simulink model "PID_finder"  (R2022b)
settings: Solver=ode4  StartTime=0.0  StopTime=30  FixedStep=0.02  RelTol=1e-3
undefined symbols (not defined in the file or in its folder): DiscIntNeverNeededParam, LQIDG_openloop_pitch, LQIDG_openloop_pitch_d, LQIDG_openloop_roll, LQIDG_openloop_roll_d
libraries: simulink_extras x2, slpidlib x2
settings Model: Creator=Ali  LastModifiedBy=Ali

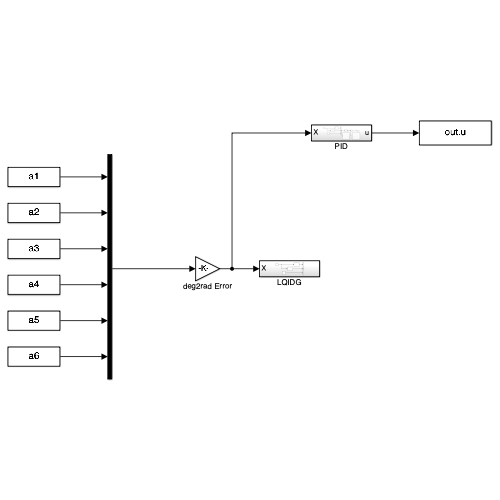
[thumbnail: Simulink's stored preview of the top-level diagram]
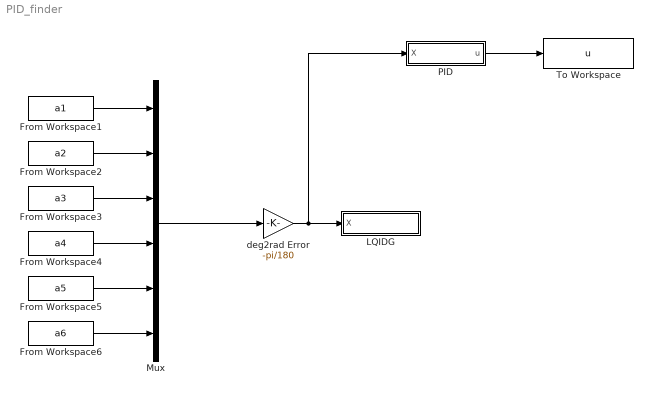
== system PID_finder ==
  From Workspace1 : FromWorkspace  VariableName=a1
  From Workspace2 : FromWorkspace  VariableName=a2
  From Workspace3 : FromWorkspace  VariableName=a3
  From Workspace4 : FromWorkspace  VariableName=a4
  From Workspace5 : FromWorkspace  VariableName=a5
  From Workspace6 : FromWorkspace  VariableName=a6
  LQIDG : Subsystem
  Mux : Mux  Inputs=6
  PID : Subsystem
  To Workspace : ToWorkspace  VariableName=u  SaveFormat=Timeseries  SampleTime=-1
  deg2rad Error : Gain  Gain=-pi/180
  wires:
  deg2rad Error/1 -> PID/1(X), LQIDG/1(X)
  Mux/1 -> deg2rad Error/1
  From Workspace1/1 -> Mux/1
  From Workspace3/1 -> Mux/3
  From Workspace2/1 -> Mux/2
  From Workspace4/1 -> Mux/4
  From Workspace5/1 -> Mux/5
  From Workspace6/1 -> Mux/6
  PID/1(u) -> To Workspace/1

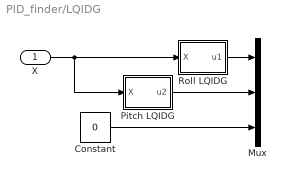
== system PID_finder/LQIDG ==
  X : Inport
  Constant : Constant  Value=0
  Mux : Mux  Inputs=3
  Pitch LQIDG : Subsystem
  Roll LQIDG : Subsystem
  wires:
  Constant/1 -> Mux/3
  Pitch LQIDG/1(u2) -> Mux/2
  X/1 -> Pitch LQIDG/1(X), Roll LQIDG/1(X)
  Roll LQIDG/1(u1) -> Mux/1

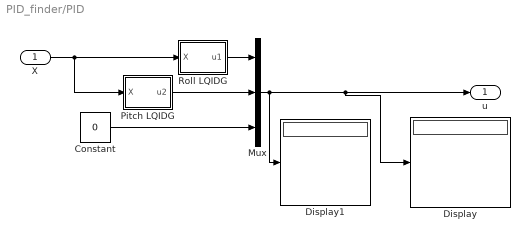
== system PID_finder/PID ==
  X : Inport
  Constant : Constant  Value=0
  Display : Display
  Display1 : Display
  Mux : Mux  Inputs=3
  Pitch LQIDG : Subsystem
  Roll LQIDG : Subsystem
  u : Outport
  wires:
  Mux/1 -> u/1, Display/1, Display1/1
  Constant/1 -> Mux/3
  Pitch LQIDG/1(u2) -> Mux/2
  X/1 -> Pitch LQIDG/1(X), Roll LQIDG/1(X)
  Roll LQIDG/1(u1) -> Mux/1

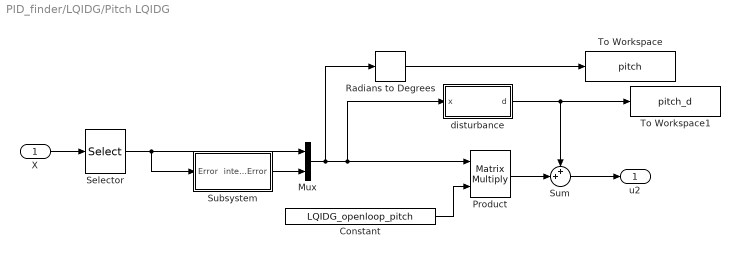
== system PID_finder/LQIDG/Pitch LQIDG ==
  X : Inport
  Constant : Constant  Value=LQIDG_openloop_pitch
  Mux : Mux  Inputs=2
  Product : Product  Multiplication=Matrix(*)
  Radians to Degrees : simulink_extras/Transformations/Radians to Degrees
  Selector : Selector  InputPortWidth=6  IndexOptions=Index vector (dialog)  Indices=[2 5]  OutputSizes=1
  Subsystem : Subsystem
  Sum : Sum  Inputs=++|
  To Workspace : ToWorkspace  VariableName=pitch  SaveFormat=Timeseries  SampleTime=-1
  To Workspace1 : ToWorkspace  VariableName=pitch_d  SaveFormat=Timeseries  SampleTime=-1
  disturbance : Subsystem
  u2 : Outport
  wires:
  Constant/1 -> Product/2
  X/1 -> Selector/1
  Subsystem/1(integ_Error) -> Mux/2
  Selector/1 -> Subsystem/1(Error), Mux/1
  Mux/1 -> Radians to Degrees/1, disturbance/1(x), Product/1
  disturbance/1(d) -> Sum/1, To Workspace1/1
  Product/1 -> Sum/2
  Sum/1 -> u2/1
  Radians to Degrees/1 -> To Workspace/1

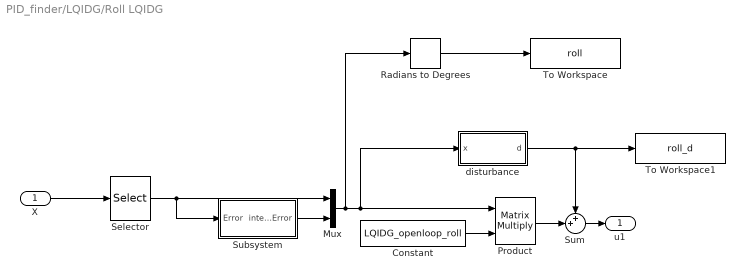
== system PID_finder/LQIDG/Roll LQIDG ==
  X : Inport
  Constant : Constant  Value=LQIDG_openloop_roll
  Mux : Mux  Inputs=2
  Product : Product  Multiplication=Matrix(*)
  Radians to Degrees : simulink_extras/Transformations/Radians to Degrees
  Selector : Selector  InputPortWidth=6  IndexOptions=Index vector (dialog)  Indices=[1 4]  OutputSizes=1
  Subsystem : Subsystem
  Sum : Sum  Inputs=++|
  To Workspace : ToWorkspace  VariableName=roll  SaveFormat=Timeseries  SampleTime=-1
  To Workspace1 : ToWorkspace  VariableName=roll_d  SaveFormat=Timeseries  SampleTime=-1
  disturbance : Subsystem
  u1 : Outport
  wires:
  Constant/1 -> Product/2
  Mux/1 -> Radians to Degrees/1, disturbance/1(x), Product/1
  X/1 -> Selector/1
  Subsystem/1(integ_Error) -> Mux/2
  Selector/1 -> Subsystem/1(Error), Mux/1
  Product/1 -> Sum/2
  Sum/1 -> u1/1
  disturbance/1(d) -> Sum/1, To Workspace1/1
  Radians to Degrees/1 -> To Workspace/1

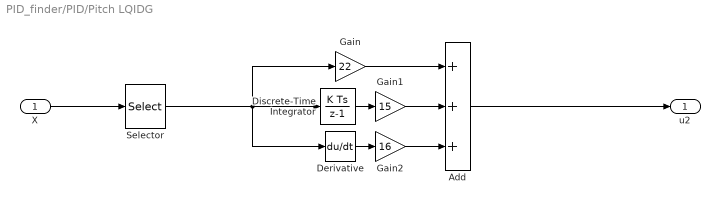
== system PID_finder/PID/Pitch LQIDG ==
  X : Inport
  Add : Sum  Inputs=+++
  Derivative : Derivative
  Discrete-Time Integrator : DiscreteIntegrator  SampleTime=-1  ICPrevOutput=DiscIntNeverNeededParam  ICPrevScaledInput=DiscIntNeverNeededParam
  Gain : Gain  Gain=22
  Gain1 : Gain  Gain=15
  Gain2 : Gain  Gain=16
  Selector : Selector  InputPortWidth=6  IndexOptions=Index vector (dialog)  Indices=[2]  OutputSizes=1
  u2 : Outport
  wires:
  X/1 -> Selector/1
  Selector/1 -> Discrete-Time Integrator/1, Gain/1, Derivative/1
  Gain1/1 -> Add/2
  Gain2/1 -> Add/3
  Discrete-Time Integrator/1 -> Gain1/1
  Derivative/1 -> Gain2/1
  Gain/1 -> Add/1
  Add/1 -> u2/1

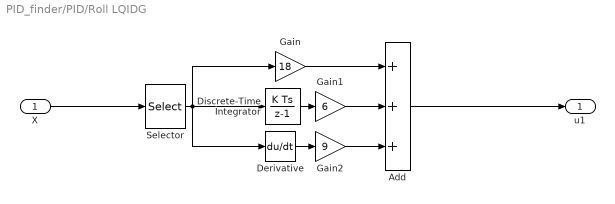
== system PID_finder/PID/Roll LQIDG ==
  X : Inport
  Add : Sum  Inputs=+++
  Derivative : Derivative
  Discrete-Time Integrator : DiscreteIntegrator  SampleTime=-1  ICPrevOutput=DiscIntNeverNeededParam  ICPrevScaledInput=DiscIntNeverNeededParam
  Gain : Gain  Gain=18
  Gain1 : Gain  Gain=6
  Gain2 : Gain  Gain=9
  Selector : Selector  InputPortWidth=6  IndexOptions=Index vector (dialog)  Indices=[1]  OutputSizes=1
  u1 : Outport
  wires:
  X/1 -> Selector/1
  Selector/1 -> Discrete-Time Integrator/1, Derivative/1, Gain/1
  Gain/1 -> Add/1
  Discrete-Time Integrator/1 -> Gain1/1
  Gain1/1 -> Add/2
  Gain2/1 -> Add/3
  Derivative/1 -> Gain2/1
  Add/1 -> u1/1

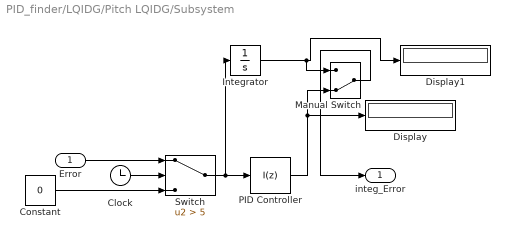
== system PID_finder/LQIDG/Pitch LQIDG/Subsystem ==
  Error : Inport
  Clock : Clock
  Constant : Constant  Value=0
  Display : Display
  Display1 : Display
  Integrator : Integrator
  Manual Switch : ManualSwitch  CurrentSetting=0
  PID Controller : slpidlib/PID Controller  Controller=I  Form=Parallel  TimeDomain=Discrete-time  UseExternalTs=off  SampleTime=-1  IntegratorMethod=Forward Euler  FilterMethod=Forward Euler  ControllerParametersSource=internal  P=1  I=1  UseKiTs=off  D=0  N=100  UseFilter=on  TunerSelectOption=Transfer Function Based (PID Tuner App)  InitialConditionSource=internal  InitialConditionForIntegrator=0.2  InitialConditionForFilter=0  DifferentiatorICPrevScaledInput=0  ExternalReset=none  TrackingMode=off  Kt=1  LimitOutput=on  SatLimitsSource=internal  UpperSaturationLimit=1.2  LowerSaturationLimit=0.2  LinearizeAsGain=on  AntiWindupMode=clamping  Kb=15  LimitIntegrator=on  UpperIntegratorSaturationLimit=1.2  LowerIntegratorSaturationLimit=0.2  POutMin=[]  POutMax=[]  IOutMin=[]  IOutMax=[]  DOutMin=[]  DOutMax=[]  NOutMin=[]  NOutMax=[]  SumOutMin=[]  SumOutMax=[]  SaturationOutMin=[]  SaturationOutMax=[]  PParamMin=[]  PParamMax=[]  IParamMin=[]  IParamMax=[]  DParamMin=[]  DParamMax=[]  NParamMin=[]  NParamMax=[]  KbParamMin=[]  KbParamMax=[]  KtParamMin=[]  KtParamMax=[]  KbOutMin=[]  KbOutMax=[]  KtOutMin=[]  KtOutMax=[]  IntegratorOutMin=[]  IntegratorOutMax=[]  FilterOutMin=[]  FilterOutMax=[]  SumI1OutMin=[]  SumI1OutMax=[]  SumI2OutMin=[]  SumI2OutMax=[]  SumI3OutMin=[]  SumI3OutMax=[]  SumI4OutMin=[]  SumI4OutMax=[]  SumDOutMin=[]  SumDOutMax=[]  DifferentiatorOutMin=[]  DifferentiatorOutMax=[]  FilterDiffOutCoefMin=[]  FilterDiffOutCoefMax=[]  ReciprocalOutMin=[]  ReciprocalOutMax=[]  SumDenOutMin=[]  SumDenOutMax=[]  SumNumOutMin=[]  SumNumOutMax=[]  DivideOutMin=[]  DivideOutMax=[]  UdiffTsProdOutMin=[]  UdiffTsProdOutMax=[]  NTsProdOutMin=[]  NTsProdOutMax=[]  UintegralTsProdOutMin=[]  UintegralTsProdOutMax=[]  UngainTsProdOutMin=[]  UngainTsProdOutMax=[]  ClampingZeroOutDataTypeStr=Inherit: Inherit via back propagation  ClampingZeroOutMin=[]  ClampingZeroOutMax=[]  FilterDenConstantOutDataTypeStr=Inherit: Inherit via back propagation  FilterDenConstantOutMin=[]  FilterDenConstantOutMax=[]  PCopyOutDataTypeStr=Inherit: Inherit via back propagation  PCopyOutMin=[]  PCopyOutMax=[]  NCopyOutDataTypeStr=Inherit: Inherit via back propagation  NCopyOutMin=[]  NCopyOutMax=[]  IntegratorContinuousStateAttributes=''  IntegratorStateMustResolveToSignalObject=off  IntegratorRTWStateStorageClass=Auto  FilterContinuousStateAttributes=''  FilterStateMustResolveToSignalObject=off  FilterRTWStateStorageClass=Auto  ParallelPVariant=Disabled  IdealPVariant=Disabled  IVariant=InternalParameters  DVariant=Disabled  IntegratorVariant=Discrete  SatVariant=Enabled  AWVariant=DiscClampingParallel  PCopyVariant=Disabled  TRVariant=Disabled  FdbkBlocksVariant=Forward  IdealPFdbkVariant=Disabled  SatFdbkVariant=Disabled  DerivativeFilterVariant=Disabled  NVariant=Disabled  NCopyVariant=Disabled_SignalSpec  FilterICVariant=Disabled  IntegratorICVariant=InternalICs  ExternalResetVariant=Disabled  TRSumVariant=Passthrough  SumFdbkVariant=Disabled  SumVariant=Passthrough_I  TsampFilterVariant=InternalTs  TsampNgainVariant=Passthrough  TsampIntegralVariant=Passthrough  ExternalSaturationOutDataTypeStr=Inherit: Same as second input
  Switch : Switch  Criteria=u2 > Threshold  Threshold=5  SaturateOnIntegerOverflow=off  InputSameDT=off
  integ_Error : Outport
  wires:
  Error/1 -> Switch/1
  Clock/1 -> Switch/2
  Switch/1 -> Integrator/1, PID Controller/1
  Constant/1 -> Switch/3
  PID Controller/1 -> Manual Switch/2, Display/1
  Integrator/1 -> Manual Switch/1, Display1/1
  Manual Switch/1 -> integ_Error/1

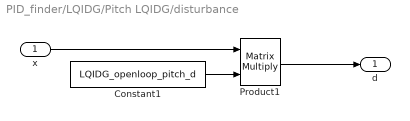
== system PID_finder/LQIDG/Pitch LQIDG/disturbance ==
  x : Inport
  Constant1 : Constant  Value=LQIDG_openloop_pitch_d
  Product1 : Product  Multiplication=Matrix(*)
  d : Outport
  wires:
  Product1/1 -> d/1
  x/1 -> Product1/1
  Constant1/1 -> Product1/2

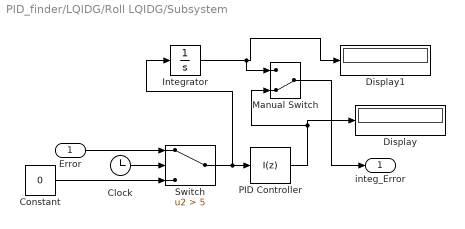
== system PID_finder/LQIDG/Roll LQIDG/Subsystem ==
  Error : Inport
  Clock : Clock
  Constant : Constant  Value=0
  Display : Display
  Display1 : Display
  Integrator : Integrator
  Manual Switch : ManualSwitch  CurrentSetting=0
  PID Controller : slpidlib/PID Controller  Controller=I  Form=Parallel  TimeDomain=Discrete-time  UseExternalTs=off  SampleTime=-1  IntegratorMethod=Forward Euler  FilterMethod=Forward Euler  ControllerParametersSource=internal  P=1  I=1  UseKiTs=off  D=0  N=100  UseFilter=on  TunerSelectOption=Transfer Function Based (PID Tuner App)  InitialConditionSource=internal  InitialConditionForIntegrator=0  InitialConditionForFilter=0  DifferentiatorICPrevScaledInput=0  ExternalReset=none  TrackingMode=off  Kt=1  LimitOutput=on  SatLimitsSource=internal  UpperSaturationLimit=1  LowerSaturationLimit=-0.2  LinearizeAsGain=on  AntiWindupMode=back-calculation  Kb=1  LimitIntegrator=on  UpperIntegratorSaturationLimit=1  LowerIntegratorSaturationLimit=-0.2  POutMin=[]  POutMax=[]  IOutMin=[]  IOutMax=[]  DOutMin=[]  DOutMax=[]  NOutMin=[]  NOutMax=[]  SumOutMin=[]  SumOutMax=[]  SaturationOutMin=[]  SaturationOutMax=[]  PParamMin=[]  PParamMax=[]  IParamMin=[]  IParamMax=[]  DParamMin=[]  DParamMax=[]  NParamMin=[]  NParamMax=[]  KbParamMin=[]  KbParamMax=[]  KtParamMin=[]  KtParamMax=[]  KbOutMin=[]  KbOutMax=[]  KtOutMin=[]  KtOutMax=[]  IntegratorOutMin=[]  IntegratorOutMax=[]  FilterOutMin=[]  FilterOutMax=[]  SumI1OutMin=[]  SumI1OutMax=[]  SumI2OutMin=[]  SumI2OutMax=[]  SumI3OutMin=[]  SumI3OutMax=[]  SumI4OutMin=[]  SumI4OutMax=[]  SumDOutMin=[]  SumDOutMax=[]  DifferentiatorOutMin=[]  DifferentiatorOutMax=[]  FilterDiffOutCoefMin=[]  FilterDiffOutCoefMax=[]  ReciprocalOutMin=[]  ReciprocalOutMax=[]  SumDenOutMin=[]  SumDenOutMax=[]  SumNumOutMin=[]  SumNumOutMax=[]  DivideOutMin=[]  DivideOutMax=[]  UdiffTsProdOutMin=[]  UdiffTsProdOutMax=[]  NTsProdOutMin=[]  NTsProdOutMax=[]  UintegralTsProdOutMin=[]  UintegralTsProdOutMax=[]  UngainTsProdOutMin=[]  UngainTsProdOutMax=[]  ClampingZeroOutDataTypeStr=Inherit: Inherit via back propagation  ClampingZeroOutMin=[]  ClampingZeroOutMax=[]  FilterDenConstantOutDataTypeStr=Inherit: Inherit via back propagation  FilterDenConstantOutMin=[]  FilterDenConstantOutMax=[]  PCopyOutDataTypeStr=Inherit: Inherit via back propagation  PCopyOutMin=[]  PCopyOutMax=[]  NCopyOutDataTypeStr=Inherit: Inherit via back propagation  NCopyOutMin=[]  NCopyOutMax=[]  IntegratorContinuousStateAttributes=''  IntegratorStateMustResolveToSignalObject=off  IntegratorRTWStateStorageClass=Auto  FilterContinuousStateAttributes=''  FilterStateMustResolveToSignalObject=off  FilterRTWStateStorageClass=Auto  ParallelPVariant=Disabled  IdealPVariant=Disabled  IVariant=InternalParameters  DVariant=Disabled  IntegratorVariant=Discrete  SatVariant=Enabled  AWVariant=BackCalculation  PCopyVariant=Disabled  TRVariant=Disabled  FdbkBlocksVariant=Forward  IdealPFdbkVariant=Disabled  SatFdbkVariant=Disabled  DerivativeFilterVariant=Disabled  NVariant=Disabled  NCopyVariant=Disabled_SignalSpec  FilterICVariant=Disabled  IntegratorICVariant=InternalICs  ExternalResetVariant=Disabled  TRSumVariant=Passthrough  SumFdbkVariant=Disabled  SumVariant=Passthrough_I  TsampFilterVariant=InternalTs  TsampNgainVariant=Passthrough  TsampIntegralVariant=Passthrough  ExternalSaturationOutDataTypeStr=Inherit: Same as second input
  Switch : Switch  Criteria=u2 > Threshold  Threshold=5  SaturateOnIntegerOverflow=off  InputSameDT=off
  integ_Error : Outport
  wires:
  Error/1 -> Switch/1
  Clock/1 -> Switch/2
  Switch/1 -> Integrator/1, PID Controller/1
  Constant/1 -> Switch/3
  PID Controller/1 -> Manual Switch/2, Display/1
  Integrator/1 -> Manual Switch/1, Display1/1
  Manual Switch/1 -> integ_Error/1

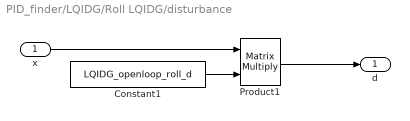
== system PID_finder/LQIDG/Roll LQIDG/disturbance ==
  x : Inport
  Constant1 : Constant  Value=LQIDG_openloop_roll_d
  Product1 : Product  Multiplication=Matrix(*)
  d : Outport
  wires:
  Product1/1 -> d/1
  x/1 -> Product1/1
  Constant1/1 -> Product1/2
